simulink model "async_sim"  (R2023b)
settings: Solver=VariableStepAuto  StartTime=0.0  StopTime=2  FixedStep=0.3  MaxStep=0.0001  RelTol=1e-3
values from neighbouring files (symbols this model uses):
  Bm = 0.02    [denklemler.m]    (also in my_params.m)
  Freq = 50    [my_params.m]
  J = 0.030    (= 0.03)    [denklemler.m]    (also in my_params.m)
  L1lr = 0.012    [denklemler.m]    (also in my_params.m)
  Lls = 0.008    [denklemler.m]    (also in my_params.m)
  Lm = 0.46    [denklemler.m]    (also in my_params.m)
  P = 2    [denklemler.m]    (also in my_params.m)
  R1r = 1.7    [my_params.m]
  Rs = 2    [denklemler.m]    (also in my_params.m)
  Vampl = 325    [my_params.m]
  w = 2*pi*Freq    (= 314.159265359)    [my_params.m]
undefined symbols (not defined in the file or in its folder): X, Y, Z
libraries: sm_lib x7, nesl_utility x3, simulink x1
settings Model: Creator=evren  LastModifiedBy=enesb
settings DataIOCC: SaveFormat=Array  SignalLogging=off  DSMLogging=off
settings DebuggingCC: ModelReferenceDataLoggingMessage=none  UnderSpecifiedDimensionMsg=warning

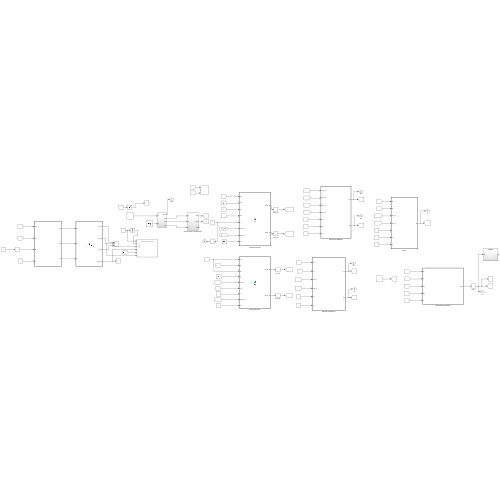
[thumbnail: Simulink's stored preview of the top-level diagram]
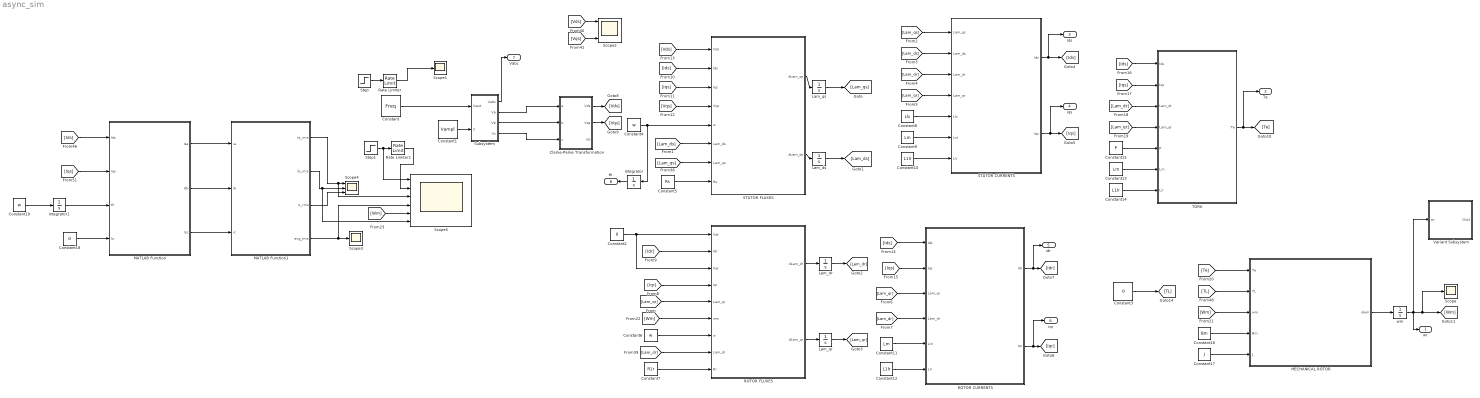
== system async_sim ==
  Clarke-Parke Transformation : Subsystem
  Constant : Constant  Value=Freq
  Constant1 : Constant  Value=Vampl
  Constant10 : Constant  Value=L1lr
  Constant11 : Constant  Value=Lm
  Constant12 : Constant  Value=L1lr
  Constant13 : Constant  Value=Lm
  Constant14 : Constant  Value=L1lr
  Constant15 : Constant  Value=P
  Constant16 : Constant  Value=Bm
  Constant17 : Constant  Value=J
  Constant18 : Constant  Value=0
  Constant19 : Constant  Value=w
  Constant2 : Constant  Value=0
  Constant3 : Constant  Value=0
  Constant4 : Constant  Value=w
  Constant5 : Constant  Value=Rs
  Constant6 : Constant  Value=w
  Constant7 : Constant  Value=R1r
  Constant8 : Constant  Value=Lls
  Constant9 : Constant  Value=Lm
  Integrator : Integrator
  Integrator1 : Integrator
  Lam_dr : Integrator
  Lam_ds : Integrator
  Lam_qr : Integrator
  Lam_qs : Integrator
  MATLAB Function : MATLAB Function  TreatAsAtomicUnit=on
  MATLAB Function1 : MATLAB Function  TreatAsAtomicUnit=on
  MECHANICAL ROTOR : MATLAB Function  TreatAsAtomicUnit=on
  "ROTOR CURRENTS " : MATLAB Function  TreatAsAtomicUnit=on
  ROTOR FLUXES : MATLAB Function  TreatAsAtomicUnit=on
  Rate Limiter : RateLimiter  RisingSlewLimit=10
  Rate Limiter1 : RateLimiter  RisingSlewLimit=0.1345  SampleTimeMode=inherited
  STATOR CURRENTS : MATLAB Function  TreatAsAtomicUnit=on
  STATOR FLUXES : MATLAB Function  TreatAsAtomicUnit=on
  Scope : Scope
  Scope1 : Scope
  Scope2 : Scope  NumInputPorts=3
  Scope3 : Scope
  Scope4 : Scope  NumInputPorts=3
  Scope5 : Scope  NumInputPorts=6
  Step : Step  After=50  SampleTime=0
  Step1 : Step  After=50  SampleTime=0
  Subsystem : Subsystem
  TORK : MATLAB Function  TreatAsAtomicUnit=on
  Variant Subsystem : Subsystem  Variant=on
  wm : Integrator  UpperSaturationLimit=100000000000000000000  LowerSaturationLimit=-100000000000000000000
  wr : Outport
  Te : Outport  Port=2
  ids : Outport  Port=3
  iqs : Outport  Port=4
  idr : Outport  Port=5
  iqr : Outport  Port=6
  Vabc : Outport  Port=7
  th : Outport  Port=8
  wires:
  Subsystem/2(Va) -> Clarke-Parke Transformation/1(a)
  Subsystem/3(Vb) -> Clarke-Parke Transformation/2(b)
  Subsystem/4(Vc) -> Clarke-Parke Transformation/3(c)
  MECHANICAL ROTOR/1(dwm) -> wm/1
  STATOR FLUXES/2(dLam_ds) -> Lam_ds/1
  ROTOR FLUXES/2(dLam_qr) -> Lam_qr/1
  STATOR FLUXES/1(dLam_qs) -> Lam_qs/1
  ROTOR FLUXES/1(dLam_dr) -> Lam_dr/1
  STATOR CURRENTS/2(Iqs) -> iqs/1, [Iqs]
  Constant2/1 -> ROTOR FLUXES/3(Vqr), ROTOR FLUXES/1(Vdr)
  Lam_qs/1 -> [Lam_qs]
  Lam_ds/1 -> [Lam_ds]
  Lam_dr/1 -> [Lam_dr]
  Lam_qr/1 -> [Lam_qr]
  [Lam_qr] -> ROTOR FLUXES/5(Lam_qr)
  [Lam_ds] -> STATOR FLUXES/6(Lam_ds)
  [Lam_qs] -> STATOR CURRENTS/1(Lam_qs)
  [Lam_qr] -> STATOR CURRENTS/4(Lam_qr)
  [Lam_ds] -> STATOR CURRENTS/2(Lam_ds)
  [Lam_dr] -> STATOR CURRENTS/3(Lam_dr)
  [Lam_qr] -> "ROTOR CURRENTS "/3(Lam_qr)
  [Lam_dr] -> "ROTOR CURRENTS "/4(Lam_dr)
  STATOR CURRENTS/1(Ids) -> ids/1, [Ids]
  "ROTOR CURRENTS "/1(Idr) -> idr/1, [Idr]
  "ROTOR CURRENTS "/2(Iqr) -> iqr/1, [Iqr]
  [Iqr] -> ROTOR FLUXES/4(Iqr)
  [Idr] -> ROTOR FLUXES/2(Idr)
  [Iqs] -> STATOR FLUXES/3(Iqs)
  [Ids] -> STATOR FLUXES/2(Ids)
  Constant4/1 -> Integrator/1, STATOR FLUXES/5(w)
  Clarke-Parke Transformation/2(Vqs) -> [Vqs]
  Clarke-Parke Transformation/1(Vds) -> [Vds]
  [Vds] -> STATOR FLUXES/1(Vds)
  [Vqs] -> STATOR FLUXES/4(Vqs)
  [Iqs] -> "ROTOR CURRENTS "/2(Iqs)
  [Ids] -> "ROTOR CURRENTS "/1(Ids)
  TORK/1(Te) -> Te/1, [Te]
  [Iqs] -> TORK/2(Iqs)
  [Ids] -> TORK/1(Ids)
  [Lam_dr] -> TORK/3(Lam_dr)
  [Lam_qr] -> TORK/4(Lam_qr)
  [Te] -> MECHANICAL ROTOR/1(Te)
  wm/1 -> Variant Subsystem/1(wr), wr/1, Scope/1, [Wm]
  [Wm] -> MECHANICAL ROTOR/3(wm)
  [Wm] -> ROTOR FLUXES/6(wm)
  Constant6/1 -> ROTOR FLUXES/7(w)
  [Lam_qs] -> STATOR FLUXES/7(Lam_qs)
  [Lam_dr] -> ROTOR FLUXES/8(Lam_dr)
  [Vds] -> Scope2/1
  [Vqs] -> Scope2/3
  Constant3/1 -> [TL]
  [TL] -> MECHANICAL ROTOR/2(TL)
  Constant5/1 -> STATOR FLUXES/8(Rs)
  Constant7/1 -> ROTOR FLUXES/9(Rr)
  Constant10/1 -> STATOR CURRENTS/7(Llr)
  Constant9/1 -> STATOR CURRENTS/6(Lm)
  Constant8/1 -> STATOR CURRENTS/5(Lls)
  Constant11/1 -> "ROTOR CURRENTS "/5(Lm)
  Constant12/1 -> "ROTOR CURRENTS "/6(Llr)
  Constant13/1 -> TORK/6(Lm)
  Constant14/1 -> TORK/7(Llr)
  Constant15/1 -> TORK/5(P)
  Constant17/1 -> MECHANICAL ROTOR/5(J)
  Constant16/1 -> MECHANICAL ROTOR/4(Bm)
  Subsystem/1(Vabc) -> Vabc/1
  Integrator/1 -> th/1
  Constant1/1 -> Subsystem/2(Input1)
  Step/1 -> Rate Limiter/1
  Rate Limiter/1 -> Scope1/1
  Step1/1 -> Rate Limiter1/1, Scope5/1
  MATLAB Function/3(Isc) -> MATLAB Function1/3(ic)
  MATLAB Function1/3(ic_rms) -> Scope4/3
  Constant19/1 -> Integrator1/1
  [Ids] -> MATLAB Function/1(Ids)
  MATLAB Function1/1(ia_rms) -> Scope5/3, Scope4/1
  [Iqs] -> MATLAB Function/2(Iqs)
  MATLAB Function/2(Isb) -> MATLAB Function1/2(ib)
  MATLAB Function1/2(ib_rms) -> Scope5/6, Scope4/2
  MATLAB Function1/4(avg_rms) -> Scope5/4, Scope3/1
  MATLAB Function/1(Isa) -> MATLAB Function1/1(ia)
  Integrator1/1 -> MATLAB Function/3(th)
  Constant18/1 -> MATLAB Function/4(Io)
  [Wm] -> Scope5/5
  Rate Limiter1/1 -> Scope5/2
  Constant/1 -> Subsystem/1(Input)

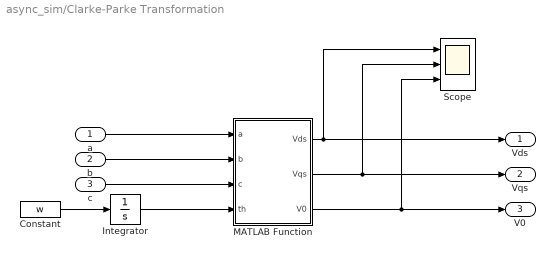
== system async_sim/Clarke-Parke Transformation ==
  a : Inport
  b : Inport  Port=2
  c : Inport  Port=3
  Constant : Constant  Value=w
  Integrator : Integrator
  MATLAB Function : MATLAB Function  TreatAsAtomicUnit=on
  Scope : Scope  NumInputPorts=3
  Vds : Outport
  Vqs : Outport  Port=2
  V0 : Outport  Port=3
  wires:
  MATLAB Function/1(Vds) -> Scope/1, Vds/1
  MATLAB Function/3(V0) -> Scope/3, V0/1
  c/1 -> MATLAB Function/3(c)
  MATLAB Function/2(Vqs) -> Scope/2, Vqs/1
  b/1 -> MATLAB Function/2(b)
  a/1 -> MATLAB Function/1(a)
  Constant/1 -> Integrator/1
  Integrator/1 -> MATLAB Function/4(th)

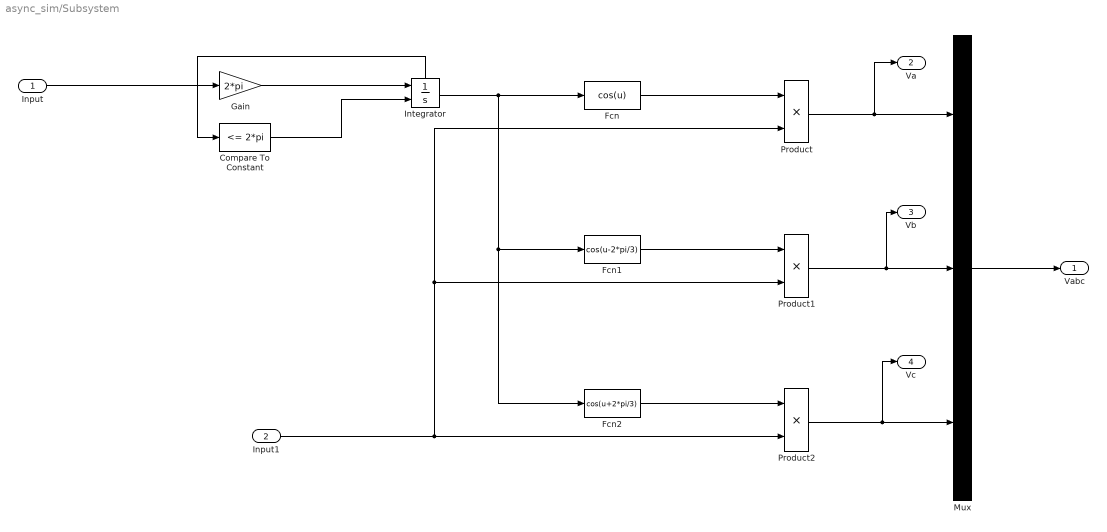
== system async_sim/Subsystem ==
  Input : Inport
  Input1 : Inport  Port=2
  Compare To Constant : simulink/Logic and Bit Operations/Compare To Constant  relop=<=  const=2*pi  OutDataTypeStr=boolean
  Fcn : Fcn  Expr=cos(u)
  Fcn1 : Fcn  Expr=cos(u-2*pi/3)
  Fcn2 : Fcn  Expr=cos(u+2*pi/3)
  Gain : Gain  Gain=2*pi
  Integrator : Integrator  ExternalReset=rising  ShowStatePort=on
  Mux : Mux  Inputs=3
  Product : Product
  Product1 : Product
  Product2 : Product
  Vabc : Outport
  Va : Outport  Port=2
  Vb : Outport  Port=3
  Vc : Outport  Port=4
  wires:
  Input1/1 -> Product2/2, Product1/2, Product/2
  Input/1 -> Gain/1
  Gain/1 -> Integrator/1
  Product2/1 -> Vc/1, Mux/3
  Integrator/State -> Compare To Constant/1
  Product1/1 -> Vb/1, Mux/2
  Integrator/1 -> Fcn2/1, Fcn1/1, Fcn/1
  Fcn/1 -> Product/1
  Product/1 -> Mux/1, Va/1
  Fcn2/1 -> Product2/1
  Fcn1/1 -> Product1/1
  Compare To Constant/1 -> Integrator/2
  Mux/1 -> Vabc/1

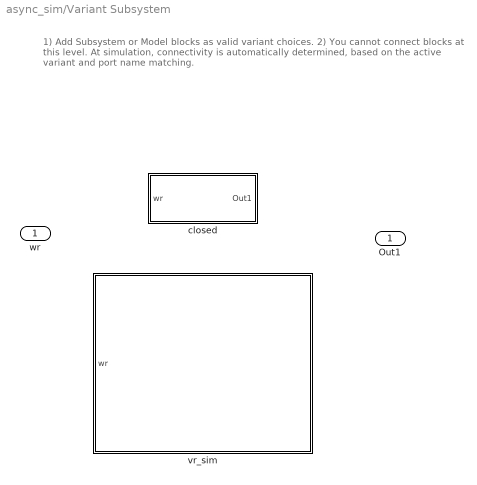
== system async_sim/Variant Subsystem ==
  note: 1) Add Subsystem or Model blocks as valid variant choices.
      | 2) You cannot connect blocks at this level. At simulation, connectivity is automatically
      | determined, based on the active variant and port name matching.
  wr : Inport
  closed : Subsystem  VariantControl=variantChoice == 0
  vr_sim : Subsystem  VariantControl=variantChoice == 1
  Out1 : Outport

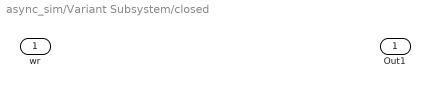
== system async_sim/Variant Subsystem/closed ==
  wr : Inport
  Out1 : Outport

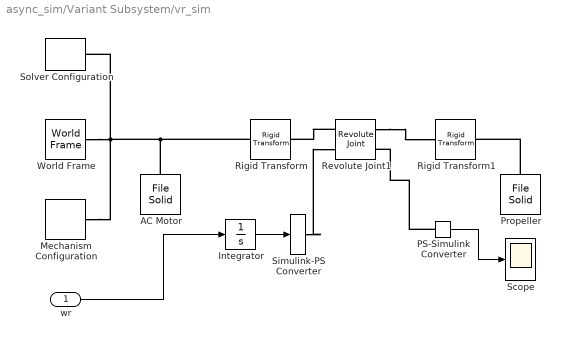
== system async_sim/Variant Subsystem/vr_sim ==
  wr : Inport
  AC Motor : sm_lib/Body Elements/File Solid  ExtGeomFileName=/home/enesb/Desktop/MKT/matlab_kodlari/proje_odevi/AC Motor.stp  UnitType=FromFile  ExtGeomFileUnits=m  StepReaderType=HEX  ExportConvexHullGeometry=off  InertiaType=CalculateFromGeometry  Mass=1  MassUnits=kg  CenterOfMass=[0 0 0]  CenterOfMassUnits=m  MomentsOfInertia=[1 1 1]  MomentsOfInertiaUnits=kg*m^2  ProductsOfInertia=[0 0 0]  ProductsOfInertiaUnits=kg*m^2  BasedOnType=Mass  Density=1000  DensityUnits=kg/m^3  DoExposeReferenceFrame=on  SerializedFrames=<Frames/>  GraphicType=FromGeometry  MarkerShape=Sphere  MarkerSize=10  GraphicVisPropType=SimpleVisualProperties  GraphicDiffuseColor=[0.6627451 0.015686275 0.19607843]  GraphicSpecularColor=[0.5 0.5 0.5 1.0]  GraphicAmbientColor=[0.15 0.15 0.15 1.0]  GraphicEmissiveColor=[0.0 0.0 0.0 1.0]  GraphicShininess=75  GraphicOpacity=1.0
  Integrator : Integrator
  Mechanism Configuration : sm_lib/Utilities/Mechanism Configuration  UniformGravity=Constant  GravityVector=[0 0 -9.80665]  GravityVectorUnits=m/s^2  LinearizationDelta=0.001  JointModeTransitionNonlinearIterations=2
  PS-Simulink Converter : nesl_utility/PS-Simulink Converter  PhysicalDomain=network_engine_domain  SubClassName=ps_output  LeftPortType=input  RightPortType=output  PseudoPeriodic=off  Frequencies=[]  VectorFormat=inherit  Unit=inherit  AffineConversion=off
  Propeller : sm_lib/Body Elements/File Solid  ExtGeomFileName=/home/enesb/Desktop/MKT/matlab_kodlari/proje_odevi/propeller.SLDPRT  UnitType=Custom  ExtGeomFileUnits=m  StepReaderType=HEX  ExportConvexHullGeometry=off  InertiaType=CalculateFromGeometry  Mass=1  MassUnits=kg  CenterOfMass=[0 0 0]  CenterOfMassUnits=m  MomentsOfInertia=[1 1 1]  MomentsOfInertiaUnits=kg*m^2  ProductsOfInertia=[0 0 0]  ProductsOfInertiaUnits=kg*m^2  BasedOnType=Mass  Density=1000  DensityUnits=kg/m^3  DoExposeReferenceFrame=on  SerializedFrames=<Frames/>  GraphicType=FromGeometry  MarkerShape=Sphere  MarkerSize=10  GraphicVisPropType=SimpleVisualProperties  GraphicDiffuseColor=[0.99215686 0.7254902 0.07058824]  GraphicSpecularColor=[0.5 0.5 0.5 1.0]  GraphicAmbientColor=[0.15 0.15 0.15 1.0]  GraphicEmissiveColor=[0.0 0.0 0.0 1.0]  GraphicShininess=75  GraphicOpacity=1.0
  Revolute Joint1 : sm_lib/Joints/Revolute Joint  JointMode=Normal  SenseConstraintForce=off  SenseConstraintForceX=off  SenseConstraintForceY=off  SenseConstraintForceZ=off  SenseConstraintTorque=off  SenseConstraintTorqueX=off  SenseConstraintTorqueY=off  SenseConstraintTorqueZ=off  SenseTotalForce=off  SenseTotalForceX=off  SenseTotalForceY=off  SenseTotalForceZ=off  SenseTotalTorque=off  SenseTotalTorqueX=off  SenseTotalTorqueY=off  SenseTotalTorqueZ=off  CompositeWrenchDir=FollowerOnBase  CompositeWrenchFrame=BaseFrame  EquilibriumPosition=0  EquilibriumPositionUnits=deg  SpringStiffness=0  SpringStiffnessUnits=N*m/deg  DampingCoefficient=0  DampingCoefficientUnits=N*m/(deg/s)  TorqueActuationMode=ComputedTorque  MotionActuationMode=InputMotion  SensePosition=off  SenseVelocity=on  SenseAcceleration=off  SenseTorqueForce=off  SenseLowerLimitTorqueForce=off  SenseUpperLimitTorqueForce=off  LowerLimitSpecify=off  LowerLimitBound=-90  LowerLimitBoundUnits=deg  LowerLimitStiffness=1e4  LowerLimitStiffnessUnits=N*m/deg  LowerLimitDamping=10  LowerLimitDampingUnits=N*m/(deg/s)  LowerLimitTransitionRegionWidth=0.1  LowerLimitTransitionRegionWidthUnits=deg  UpperLimitSpecify=off  UpperLimitBound=90  UpperLimitBoundUnits=deg  UpperLimitStiffness=1e4  UpperLimitStiffnessUnits=N*m/deg  UpperLimitDamping=10  UpperLimitDampingUnits=N*m/(deg/s)  UpperLimitTransitionRegionWidth=0.1  UpperLimitTransitionRegionWidthUnits=deg  PositionTargetSpecify=off  PositionTargetPriority=High  PositionTargetValue=0  PositionTargetValueUnits=deg  VelocityTargetSpecify=off  VelocityTargetPriority=High  VelocityTargetValue=0  VelocityTargetValueUnits=deg/s
  Rigid Transform : sm_lib/Frames and Transforms/Rigid Transform  TranslationMethod=None  TranslationStandardOffset=0  TranslationStandardOffsetUnits=m  TranslationStandardAxis=+Z  TranslationCartesianOffset=[0 0 0]  TranslationCartesianOffsetUnits=m  TranslationROffset=0  TranslationROffsetUnits=m  TranslationZOffset=0  TranslationZOffsetUnits=m  TranslationThetaOffset=0  TranslationThetaOffsetUnits=deg  RotationMethod=StandardAxis  RotationAngleUnits=deg  RotationStandardAxis=+X  RotationAngle=90  RotationArbitraryAxis=[0 0 1]  FollAlignAxisA=+X  BaseAlignAxisA=+Y  FollAlignAxisB=+Y  BaseAlignAxisB=+Z  RotationSequenceAxes=FollowerAxes  RotationSequence=XYX  RotationSequenceAngles=[0 0 0]  RotationSequenceAnglesUnits=deg  RotationMatrix=[1 0 0; 0 1 0; 0 0 1]  Quaternion=[1 0 0 0]
  Rigid Transform1 : sm_lib/Frames and Transforms/Rigid Transform  TranslationMethod=StandardAxis  TranslationStandardOffset=7  TranslationStandardOffsetUnits=cm  TranslationStandardAxis=+Z  TranslationCartesianOffset=[0 0 0]  TranslationCartesianOffsetUnits=m  TranslationROffset=0  TranslationROffsetUnits=m  TranslationZOffset=0  TranslationZOffsetUnits=m  TranslationThetaOffset=0  TranslationThetaOffsetUnits=deg  RotationMethod=None  RotationAngleUnits=deg  RotationStandardAxis=+Z  RotationAngle=0.0  RotationArbitraryAxis=[0 0 1]  FollAlignAxisA=+X  BaseAlignAxisA=+Y  FollAlignAxisB=+Y  BaseAlignAxisB=+Z  RotationSequenceAxes=FollowerAxes  RotationSequence=XYX  RotationSequenceAngles=[0 0 0]  RotationSequenceAnglesUnits=deg  RotationMatrix=[1 0 0; 0 1 0; 0 0 1]  Quaternion=[1 0 0 0]
  Scope : Scope
  Simulink-PS Converter : nesl_utility/Simulink-PS Converter  PhysicalDomain=network_engine_domain  SubClassName=ps_input  LeftPortType=input  RightPortType=output  PseudoPeriodic=off  Frequencies=[]  NoiseDistribution=none  NoiseParameters=[]  Unit=1  AffineConversion=off  FilteringAndDerivatives=filter  SimscapeFilterOrder=2  InputFilterTimeConstant=0.001  UdotUserProvided=0
  Solver Configuration : nesl_utility/Solver Configuration  PhysicalDomain=network_engine_domain  SubClassName=solver  LeftPortType=input  RightPortType=generic  Tones=[]  Harmonics=[]  SimulateNoise=off  Profile=off  UseLocalSampling=off  EnableSwitchedLinearOptims=on  FrequencyDomain=off  UseCCode=off  RelTol=0.001  AbsTol=1e-06  MinStep=1e-09  ToWorkspace=off  RevertToSquareIcSolve=off  NumHomotopyIterations=100  PhasorMode=off  PhasorModeNumHarmonics=1  ConsistencySolver=NEWTON_XTOL_AFTER_FTOL  IndexReductionMethod=DerivativeReplacement  DoDC=off  ResidualTolerance=1e-09  ConsistencyTolSource=GLOBAL  ConsistencyAbsTol=0.001  ConsistencyRelTol=0.001  ConsistencyTolFactor=0.001  UseLocalSolver=off  LocalSolverChoice=NE_BACKWARD_EULER_ADVANCER  ResolveIndetEquations=on  FunctionEvalNumThread=1  LocalSolverSampleTime=0.001  DoFixedCost=off  MaxNonlinIter=3  MaxModeIter=2  ComputeImpulses=off  ImpulseIterations=2  LinearAlgebra=Sparse  LinearAlgebraNumThread=0  EquationFormulation=NE_TIME_EF  DelaysMemoryBudget=1024  AutomaticFiltering=on  FilteringTimeConstant=0.001  PartitionStorageMethod=AS_NEEDED  PartitionMemoryBudget=1024  PartitionMethod=FAST  MultibodyUseLocalSolver=off  MultibodyLocalSolverChoice=ODE1  MultibodyLocalSolverSampleTime=0.001
  World Frame : sm_lib/Frames and Transforms/World Frame
  wires:
  PS-Simulink Converter/1 -> Scope/1
  Integrator/1 -> Simulink-PS Converter/1
  wr/1 -> Integrator/1
  connections:
  Revolute Joint1/LConn1 -- Rigid Transform/RConn1
  Solver Configuration/RConn1 -- Rigid Transform/LConn1 -- AC Motor/RConn1 -- World Frame/RConn1 -- Mechanism Configuration/RConn1
  Propeller/RConn1 -- Rigid Transform1/RConn1
  Revolute Joint1/RConn1 -- Rigid Transform1/LConn1
  Simulink-PS Converter/RConn1 -- Revolute Joint1/LConn2
  PS-Simulink Converter/LConn1 -- Revolute Joint1/RConn2

== matlab function async_sim/MECHANICAL ROTOR ==
  data: Te input; dwm output; TL input; wm input; Bm input; J input
function dwm = fcn(Te, TL, wm, Bm, J)



dwm = (Te - (Bm*wm) -TL)/J;

== matlab function async_sim/MATLAB Function ==
  data: Ids input; Isa output; Iqs input; th input; Isb output; Io input; Isc output
function [Isa, Isb, Isc] = fcn(Ids, Iqs, th, Io)



M = (3/2)*[cos(th), sin(th), 1;
     cos(th-2*pi/3), sin(th-2*pi/3), 1;
     cos(th+2*pi/3), sin(th+2*pi/3), 1];

I = [Ids; Iqs; Io];

x = M*I;

Isa = x(1);

Isb = x(2);

Isc = x(3);

== matlab function async_sim/MATLAB Function1 ==
  data: ia input; ia_rms output; ib input; ic input; ib_rms output; ic_rms output; avg_rms output
function [ia_rms, ib_rms, ic_rms, avg_rms] = calculateRMS(ia, ib, ic)
% Bu fonksiyon üç fazlı akımın RMS değerlerini hesaplar.

% RMS hesaplama
ia_rms = sqrt(mean(ia.^2));
ib_rms = sqrt(mean(ib.^2));
ic_rms = sqrt(mean(ic.^2));

% Ortalama RMS değeri
avg_rms = mean([ia_rms, ib_rms, ic_rms]);
end

== matlab function async_sim/STATOR FLUXES ==
  data: Vds input; Ids input; Iqs input; Vqs input; dLam_qs output; w input; dLam_ds output; Lam_ds input; Lam_qs input; Rs input
function [dLam_qs, dLam_ds]  = fcn(Vds, Ids, Iqs, Vqs, w, Lam_ds, Lam_qs, Rs)




dLam_qs = Vqs - Rs*Iqs - w*(Lam_ds);

dLam_ds = Vds - Rs*Ids + w*(Lam_qs);

== matlab function async_sim/Clarke-Parke Transformation/MATLAB Function ==
  data: a input; Vds output; b input; c input; th input; Vqs output; V0 output
function [Vds, Vqs, V0] = fcn(a, b, c, th)

 %x1 =  [Vd; Vq; V0];

 x2 =  (2/3)*[cos(th), cos(th-2*pi/3), cos(th+2*pi/3);
        sin(th), sin(th-2*pi/3), sin(th+2*pi/3);
        1/2, 1/2, 1/2];
 %x2 =  (2/3)*[1, -1/2, -1/2;0,sqrt(3)/2,-sqrt(3)/2 ;1/2, 1/2, 1/2];

 x3 =  [a;b;c];

 x4 = x2 * x3;
 
Vds = x4(1);
Vqs = x4(2);
V0 = x4(3);

== matlab function async_sim/ROTOR FLUXES ==
  data: Vdr input; dLam_dr output; Idr input; Vqr input; Iqr input; Lam_qr input; wm input; dLam_qr output; w input; Lam_dr input; Rr input
function [dLam_dr, dLam_qr] = fcn(Vdr, Idr, Vqr, Iqr, Lam_qr, wm, w, Lam_dr, Rr)






dLam_dr = Vdr - (Rr*Idr) + (w - wm)*(Lam_qr);

dLam_qr = Vqr - (Rr*Iqr) - (w - wm)*(Lam_dr);

== matlab function async_sim/STATOR CURRENTS ==
  data: Lam_qs input; Lam_ds input; Ids output; Lam_dr input; Lam_qr input; Iqs output; Lls input; Lm input; Llr input
function [Ids, Iqs] = fcn(Lam_qs, Lam_ds, Lam_dr, Lam_qr, Lls, Lm, Llr)




Lr = Llr + Lm;
Ls = Lls + Lm;



Iqs = ((Lr*Lam_qs)-(Lm*Lam_qr))/((Lr*Ls)-(Lm^2));

Ids = ((Lr*Lam_ds)-(Lm*Lam_dr))/((Lr*Ls)-(Lm^2));

== matlab function async_sim/ROTOR CURRENTS  ==
  data: Ids input; Iqs input; Lam_qr input; Lam_dr input; Idr output; Iqr output; Lm input; Llr input
function [Idr, Iqr] = fcn(Ids, Iqs, Lam_qr, Lam_dr, Lm, Llr)




Lr = Llr + Lm;





Idr = (Lam_dr - (Lm*Ids))/Lr;

Iqr = (Lam_qr - (Lm*Iqs))/Lr;

== matlab function async_sim/TORK ==
  data: Ids input; Te output; Iqs input; Lam_dr input; Lam_qr input; P input; Lm input; Llr input
function Te = fcn(Ids, Iqs, Lam_dr, Lam_qr, P, Lm, Llr)




Lr = Llr + Lm;


Te = (3*P*Lm*((Lam_dr*Iqs)-(Lam_qr*Ids)))/(4*Lr);
